simulink model "modelo_pid_lambda_autogen"  (R2025b)
settings: Solver=ode45  StartTime=0.0  StopTime=t_stop  RelTol=1e-3
values from neighbouring files (symbols this model uses):
  Gc_den = conv([tau_i 0], [tau_f 1])    [pid_lambda_simulink.m]
  Gc_num = Kc * [tau_i * tau_d tau_i 1]    [pid_lambda_simulink.m]
  Gp_den = conv([15 1], [3 1])    [pid_lambda_simulink.m]
  Gp_num = [-9 1]    [pid_lambda_simulink.m]
  r_step = 1    [pid_lambda_simulink.m]
settings Model: Creator=sergioe.ropero  LastModifiedBy=sergioe.ropero

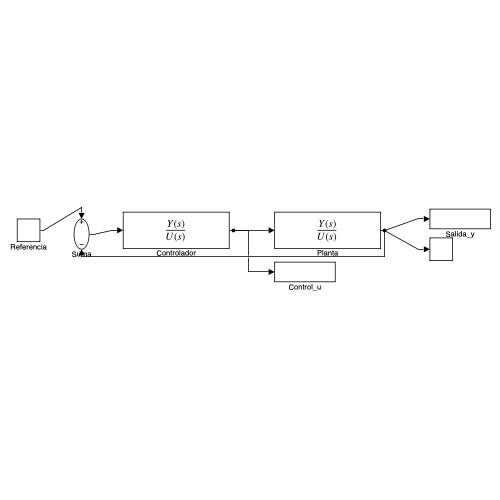
[thumbnail: Simulink's stored preview of the top-level diagram]
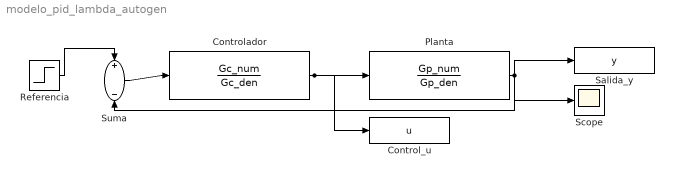
== system modelo_pid_lambda_autogen ==
  Control_u : ToWorkspace  VariableName=u  SaveFormat=Timeseries  SampleTime=-1
  Controlador : TransferFcn  Numerator=Gc_num  Denominator=Gc_den
  Planta : TransferFcn  Numerator=Gp_num  Denominator=Gp_den
  Referencia : Step  Time=0  After=r_step  SampleTime=0
  Salida_y : ToWorkspace  VariableName=y  SaveFormat=Timeseries  SampleTime=-1
  Scope : Scope
  Suma : Sum  Inputs=+-
  wires:
  Referencia/1 -> Suma/1
  Suma/1 -> Controlador/1
  Controlador/1 -> Planta/1, Control_u/1
  Planta/1 -> Salida_y/1, Scope/1, Suma/2
